simulink model "Simulation_with_controller"  (R2017a)
settings: Solver=VariableStepAuto  StartTime=0.0  StopTime=10.0  RelTol=1e-3
settings Model: Creator=Syahmi  LastModifiedBy=Syahmi

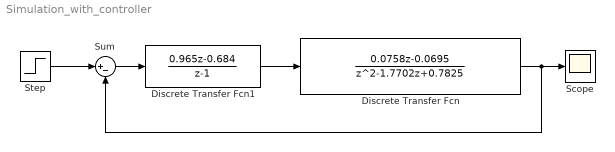
== system Simulation_with_controller ==
  Discrete Transfer Fcn : DiscreteTransferFcn  Numerator=[0.0758 -0.0695]  Denominator=[1 -1.7702 0.7825]
  Discrete Transfer Fcn1 : DiscreteTransferFcn  Numerator=[0.965 -0.684]  Denominator=[1 -1]
  Scope : Scope
  Step : Step  SampleTime=0
  Sum : Sum  Inputs=|+-
  wires:
  Discrete Transfer Fcn/1 -> Sum/2, Scope/1
  Step/1 -> Sum/1
  Sum/1 -> Discrete Transfer Fcn1/1
  Discrete Transfer Fcn1/1 -> Discrete Transfer Fcn/1
